simulink subsystem "BearingDynamicsSingleAxis"  (R2021b)
settings: Solver=VariableStepAuto  StartTime=0.0  StopTime=10.0  RelTol=1e-3
values from neighbouring files (symbols this model uses):
  cEHD = 1376.8    [V8_tunedParameters.mat]
  cp = 2210.7    [V8_tunedParameters.mat]
  cr = 9424.8    [V8_tunedParameters.mat]
  cs = 1376.8    [V8_tunedParameters.mat]
  kp = 151000000    [V8_tunedParameters.mat]
  kr = 1141000000    [V8_tunedParameters.mat]
  ks = 74200000    [V8_tunedParameters.mat]
  mi = 25.65    [V8_tunedParameters.mat]
  mo = 12.638    [V8_tunedParameters.mat]
  mr = 1    [V8_tunedParameters.mat]
settings Model: Creator=PhilippSchildt  LastModifiedBy=PhilippSchildt
settings SolverCC: AlgebraicLoopSolver=TrustRegion
settings DebuggingCC: SFMachineParentedDataDiag=warning

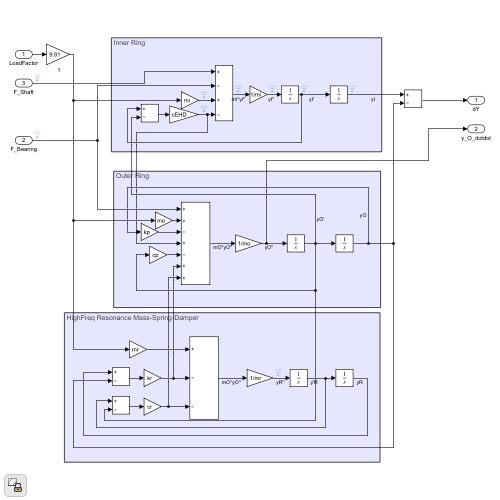
[thumbnail: Simulink's stored preview of the top-level diagram]
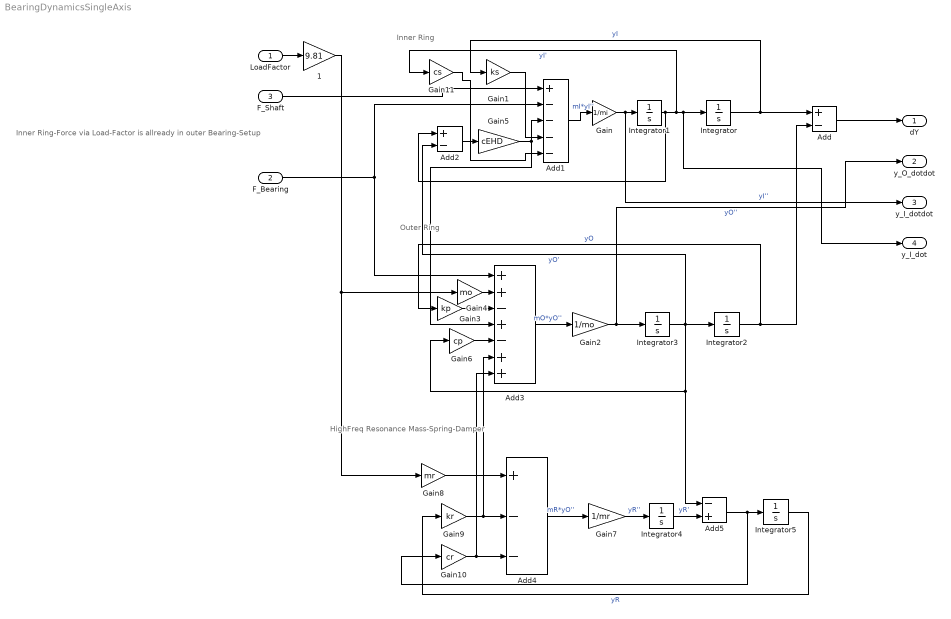
== system BearingDynamicsSingleAxis ==
  note: Inner Ring-Force via Load-Factor is allready in outer Bearing-Setup
  note: Outer Ring
  note: Inner Ring
  note: HighFreq Resonance Mass-Spring-Damper
  LoadFactor : Inport
  F_Bearing : Inport  Port=2
  F_Shaft : Inport  Port=3
  " 1" : Gain  Gain=9.81
  Add : Sum  Inputs=+-
  Add1 : Sum  Inputs=+----
  Add2 : Sum  Inputs=+-
  Add3 : Sum  Inputs=++-+-++
  Add4 : Sum  Inputs=+--
  Add5 : Sum  Inputs=-+
  Gain : Gain  Gain=1/mi
  Gain1 : Gain  Gain=ks
  Gain10 : Gain  Gain=cr
  Gain11 : Gain  Gain=cs
  Gain2 : Gain  Gain=1/mo
  Gain3 : Gain  Gain=mo
  Gain4 : Gain  Gain=kp
  Gain5 : Gain  Gain=cEHD
  Gain6 : Gain  Gain=cp
  Gain7 : Gain  Gain=1/mr
  Gain8 : Gain  Gain=mr
  Gain9 : Gain  Gain=kr
  Integrator : Integrator
  Integrator1 : Integrator
  Integrator2 : Integrator
  Integrator3 : Integrator  InitialCondition=1e-5
  Integrator4 : Integrator  InitialCondition=1e-5
  Integrator5 : Integrator  InitialCondition=1e-5
  dY : Outport
  y_O_dotdot : Outport  Port=2
  y_I_dotdot : Outport  Port=3
  y_I_dot : Outport  Port=4
  wires:
  Gain11/1 -> Add1/5
  Gain1/1 -> Add1/4
  Gain10/1 -> Add3/7, Add4/3
  Gain9/1 -> Add3/6, Add4/2
  Gain8/1 -> Add4/1
  Add4/1 -> Gain7/1  "mR*yO''"
  Integrator5/1 -> Gain9/1  "yR"
  Gain7/1 -> Integrator4/1  "yR''"
  LoadFactor/1 -> " 1"/1
  Integrator/1 -> Gain1/1, Add/1  "yI"
  Integrator1/1 -> Add2/1, Gain11/1, Integrator/1, y_I_dot/1  "yI'"
  Gain/1 -> y_I_dotdot/1, Integrator1/1  "yI''"
  Add1/1 -> Gain/1  "mI*yI''"
  F_Shaft/1 -> Add1/1
  F_Bearing/1 -> Add1/2, Add3/1
  " 1"/1 -> Gain8/1, Gain3/1
  Integrator3/1 -> Gain6/1, Add5/1, Integrator2/1, Add2/2  "yO'"
  Integrator2/1 -> Add/2, Gain4/1  "yO"
  Gain2/1 -> Integrator3/1, y_O_dotdot/1  "yO''"
  Add3/1 -> Gain2/1  "mO*yO''"
  Gain3/1 -> Add3/2
  Gain4/1 -> Add3/3
  Gain5/1 -> Add3/4, Add1/3
  Add2/1 -> Gain5/1
  Gain6/1 -> Add3/5
  Add/1 -> dY/1
  Add5/1 -> Integrator5/1, Gain10/1
  Integrator4/1 -> Add5/2  "yR'"
